simulink model "modeloRobot"  (R2018b)
settings: Solver=VariableStepAuto  StartTime=0.0  StopTime=10.0  RelTol=1e-3
settings Model: Creator=mite0  LastModifiedBy=mite0

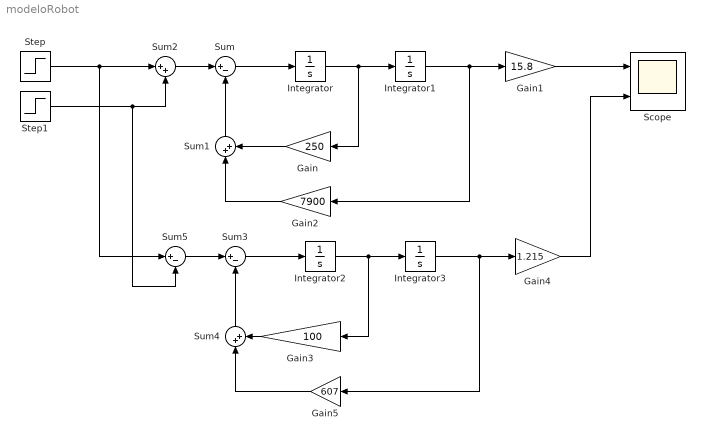
== system modeloRobot ==
  Gain : Gain  Gain=250
  Gain1 : Gain  Gain=15.8
  Gain2 : Gain  Gain=7900
  Gain3 : Gain  Gain=100
  Gain4 : Gain  Gain=1.215
  Gain5 : Gain  Gain=607
  Integrator{,1..3} (4 alike) : Integrator
  Scope : Scope  NumInputPorts=2
  Step : Step  After=0  SampleTime=0
  Step1 : Step  After=100  SampleTime=0
  Sum : Sum  Inputs=|+-
  Sum1 : Sum  Inputs=|++
  Sum2 : Sum  Inputs=|++
  Sum3 : Sum  Inputs=|+-
  Sum4 : Sum  Inputs=|++
  Sum5 : Sum  Inputs=|+-
  wires:
  Sum/1 -> Integrator/1
  Sum1/1 -> Sum/2
  Gain/1 -> Sum1/2
  Integrator/1 -> Gain/1, Integrator1/1
  Gain2/1 -> Sum1/1
  Integrator1/1 -> Gain2/1, Gain1/1
  Gain1/1 -> Scope/1
  Sum2/1 -> Sum/1
  Sum5/1 -> Sum3/1
  Sum3/1 -> Integrator2/1
  Sum4/1 -> Sum3/2
  Step1/1 -> Sum5/2, Sum2/2
  Gain4/1 -> Scope/2
  Integrator2/1 -> Gain3/1, Integrator3/1
  Gain5/1 -> Sum4/1
  Integrator3/1 -> Gain5/1, Gain4/1
  Step/1 -> Sum5/1, Sum2/1
  Gain3/1 -> Sum4/2
